simulink model "ex1modeling"  (R2021b)
settings: Solver=VariableStepAuto  StartTime=0.0  StopTime=100  RelTol=1e-3
libraries: spsSeriesRLCBranchLib x4, spsVoltageMeasurementLib x2, spsControlledVoltageSourceLib x1, simulink x1, simulink_extras x1, spspowerguiLib x1
settings Model: Creator=dhan  LastModifiedBy=dhan

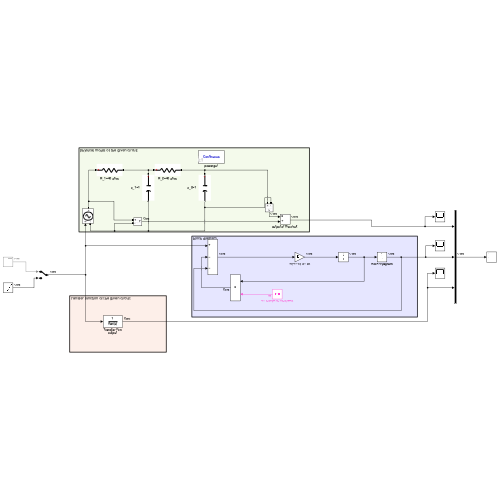
[thumbnail: Simulink's stored preview of the top-level diagram]
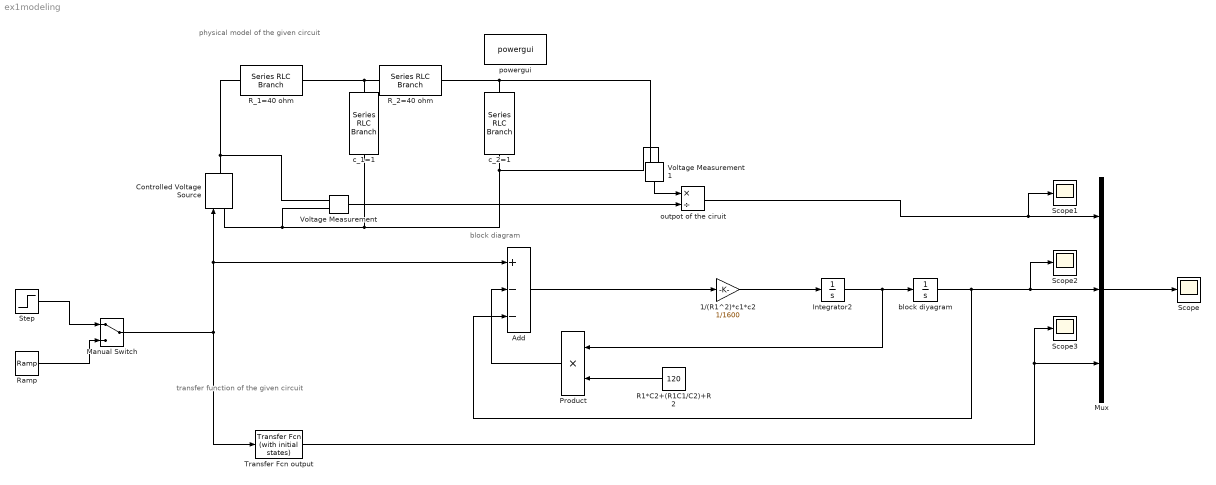
== system ex1modeling ==
  note: transfer function of the given circuit
  note: physical model of the given circuit
  note: block diagram
  1/(R1^2)*c1*c2 : Gain  Gain=1/1600
  Add : Sum  Inputs=+--
  Controlled Voltage Source : spsControlledVoltageSourceLib/Controlled Voltage Source  Initialize=on  Source_Type=AC  Amplitude=0  Phase=0  Frequency=0  Measurements=None
  Integrator2 : Integrator
  Manual Switch : ManualSwitch
  Mux : Mux  Inputs=3
  Product : Product
  R1*C2+(R1C1/C2)+R2 : Constant  Value=120
  R_1=40 ohm : spsSeriesRLCBranchLib/Series RLC Branch  LConnTagsString=__new0  RConnTagsString=__new0  BranchType=R  Resistance=40  Inductance=1e-3  SetiL0=off  InitialCurrent=0  Capacitance=1e-6  Setx0=off  InitialVoltage=0  Measurements=None
  R_2=40 ohm : spsSeriesRLCBranchLib/Series RLC Branch  LConnTagsString=__new0  RConnTagsString=__new0  BranchType=R  Resistance=40  Inductance=1e-3  SetiL0=off  InitialCurrent=0  Capacitance=1e-6  Setx0=off  InitialVoltage=0  Measurements=None
  Ramp : simulink/Sources/Ramp  slope=1  start=0  InitialOutput=0
  Scope{,1..3} (4 alike) : Scope
  Step : Step  SampleTime=0
  Transfer Fcn output : simulink_extras/Additional Linear/Transfer Fcn (with initial states)  N=[1]  D=[1600 120 1]  X0=1
  Voltage Measurement : spsVoltageMeasurementLib/Voltage Measurement  PhasorSimulation=off  OutputType=Complex  PSBequivalent=0
  Voltage Measurement1 : spsVoltageMeasurementLib/Voltage Measurement  PhasorSimulation=off  OutputType=Complex  PSBequivalent=0
  block diyagram : Integrator
  c_1=1 : spsSeriesRLCBranchLib/Series RLC Branch  LConnTagsString=__new0  RConnTagsString=__new0  BranchType=C  Resistance=1  Inductance=1e-3  SetiL0=off  InitialCurrent=0  Capacitance=1  Setx0=off  InitialVoltage=0  Measurements=None
  c_2=1 : spsSeriesRLCBranchLib/Series RLC Branch  LConnTagsString=__new0  RConnTagsString=__new0  BranchType=C  Resistance=1  Inductance=1e-3  SetiL0=off  InitialCurrent=0  Capacitance=1  Setx0=off  InitialVoltage=0  Measurements=None
  "outpot of the ciruit " : Product  Inputs=*/
  powergui : spspowerguiLib/powergui  Priority=1  SimulationMode=Continuous  SampleTime=50e-6  frequency=60  Iterations=50  frequencyindice=0  Pbase=100e6  ErrMax=1e-4  UnitsV=kV  UnitsW=MW  buscounter=0  FunctionMessages=off  echomessages=off  EnableUseOfTLC=off  CurrentSourceSwitches=off  DisableSnubberDevices=off  DisableRonSwitches=off  DisableVfSwitches=off  DisplayEquations=off  AutomaticDiscreteSolvers=off  SolverType=Tustin/Backward Euler (TBE)  Interpol=off  ExternalGateDelay=off  methode=off  Ts=100  x0status=blocks  SPID=on  SwTol=0  HookPort=off  NonlinearTolerance=1e-4  nMaxIteration=100  ContinueOnMaxIteration=off  RestoreLinks=warning  ResistiveCurrentMeasurement=off  Frange=[0:2:500]  Ylog=off  Xlog=on  ShowGrid=off  save=off  variable=ZData  structure=0  ZoomFFT=off  StartTime=0.0  cycles=1  DisplayStyle=1  fundamental=60  FreqAxis=off  MaxFrequency=1000  frequencyindicesteady=1  RmsSteady=1  display=off
  wires:
  Ramp/1 -> Manual Switch/2
  Step/1 -> Manual Switch/1
  Manual Switch/1 -> Controlled Voltage Source/1, Add/1, Transfer Fcn output/1
  Voltage Measurement1/1 -> "outpot of the ciruit "/1
  Voltage Measurement/1 -> "outpot of the ciruit "/2
  Transfer Fcn output/1 -> Mux/3, Scope3/1
  Mux/1 -> Scope/1
  "outpot of the ciruit "/1 -> Scope1/1, Mux/1
  Add/1 -> 1/(R1^2)*c1*c2/1
  Integrator2/1 -> Product/1, block diyagram/1
  1/(R1^2)*c1*c2/1 -> Integrator2/1
  Product/1 -> Add/2
  block diyagram/1 -> Scope2/1, Mux/2, Add/3
  R1*C2+(R1C1/C2)+R2/1 -> Product/2
  connections:
  Controlled Voltage Source/RConn1 -- Voltage Measurement/LConn1 -- R_1=40 ohm/LConn1
  R_1=40 ohm/RConn1 -- R_2=40 ohm/LConn1 -- c_1=1/LConn1
  c_2=1/RConn1 -- Voltage Measurement1/LConn2 -- c_1=1/RConn1 -- Voltage Measurement/LConn2 -- Controlled Voltage Source/LConn1
  R_2=40 ohm/RConn1 -- Voltage Measurement1/LConn1 -- c_2=1/LConn1
